simulink model "RiggsIodine"  (R2023a)
settings: Solver=VariableStepAuto  StartTime=0.0  StopTime=300  RelTol=1e-3
libraries: simulink x1

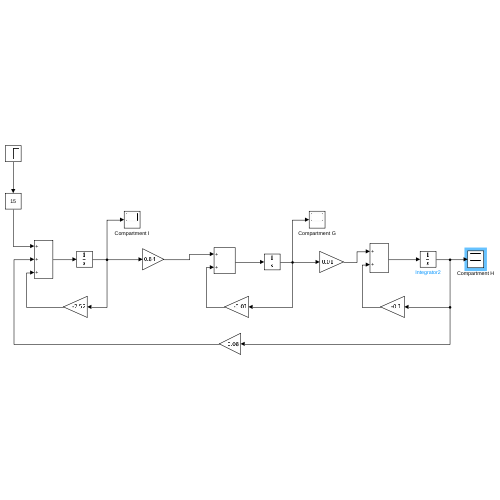
[thumbnail: Simulink's stored preview of the top-level diagram]
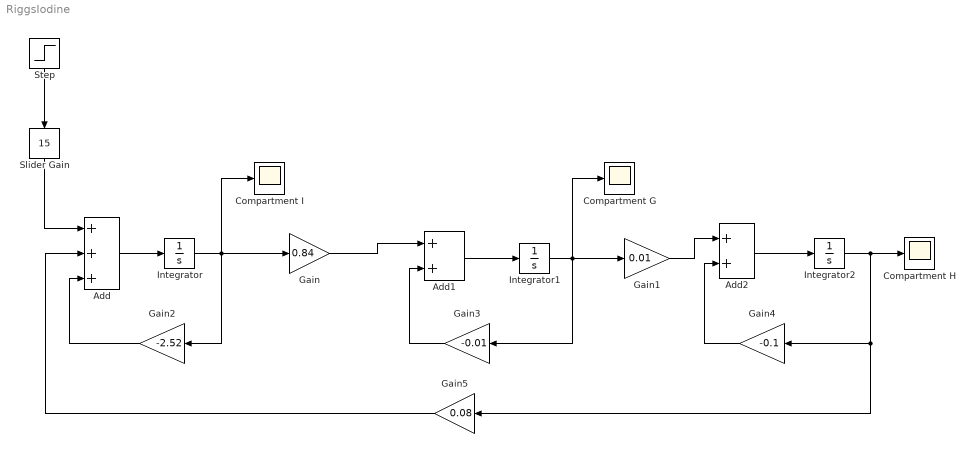
== system RiggsIodine ==
  Add : Sum  Inputs=+++
  Add1 : Sum
  Add2 : Sum
  Compartment G : Scope
  Compartment H : Scope
  Compartment I : Scope
  Gain : Gain  Gain=0.84
  Gain1 : Gain  Gain=0.01
  Gain2 : Gain  Gain=-2.52
  Gain3 : Gain  Gain=-0.01
  Gain4 : Gain  Gain=-0.1
  Gain5 : Gain  Gain=0.08
  Integrator : Integrator  InitialCondition=81.2
  Integrator1 : Integrator  InitialCondition=6821
  Integrator2 : Integrator  InitialCondition=682
  Slider Gain : simulink/Math Operations/Slider Gain  gain=15  low=0  high=20
  Step : Step  Time=0  SampleTime=0
  wires:
  Step/1 -> Slider Gain/1
  Slider Gain/1 -> Add/1
  Add/1 -> Integrator/1
  Integrator/1 -> Gain2/1, Compartment I/1, Gain/1
  Gain/1 -> Add1/1
  Add1/1 -> Integrator1/1
  Integrator1/1 -> Gain3/1, Compartment G/1, Gain1/1
  Gain1/1 -> Add2/1
  Gain4/1 -> Add2/2
  Gain3/1 -> Add1/2
  Add2/1 -> Integrator2/1
  Integrator2/1 -> Compartment H/1, Gain5/1, Gain4/1
  Gain5/1 -> Add/2
  Gain2/1 -> Add/3
